simulink model "Six_DOF"  (R2018b)
settings: Solver=FixedStepAuto  StartTime=0.0  StopTime=1000  FixedStep=1/90  MaxStep=2.0  RelTol=1e-3
InitFcn:
  | initializeVariables
StopFcn:
  | postProcessResults
values from neighbouring files (symbols this model uses):
  airplane =     [Airplane.mat]    (also in POC_airplane.mat; POC_test.mat; calculateForces.m = A.airplane; cl_test2.m = A.airplane)
  m = 3000    [InerGeo.mat]    (also in calculateForces.m = [Cl;Cm;Cn]*(0.5*rho*Vinf^2*S*cbar); initializeVariables.m = airplane.weights.MTOW)
undefined symbols (not defined in the file or in its folder): ft, s
libraries: simulink_extras x14, aerolibconvert2 x5, simulink x5, aerolibasang x4, aerolibanimutils x2, shared6dof x1, aerolibfltsims x1, dspstat3 x1
settings Model: Creator=Devansh  LastModifiedBy=jmzg1
settings DebuggingCC: ReadBeforeWriteMsg=DisableAll  WriteAfterWriteMsg=DisableAll  WriteAfterReadMsg=DisableAll  MultiTaskDSMMsg=none
settings HardwareCC: ProdBitPerLong=64  ProdHWDeviceType=Intel->x86-64 (Mac OS X)
settings ModelReferenceCC: UpdateModelReferenceTargets=IfOutOfDate
settings SFSimCC: SFSimEcho=off  SimUseLocalCustomCode=off
settings RTWCC: RTWUseLocalCustomCode=off
settings CodeAppCC: StateflowObjectComments=on

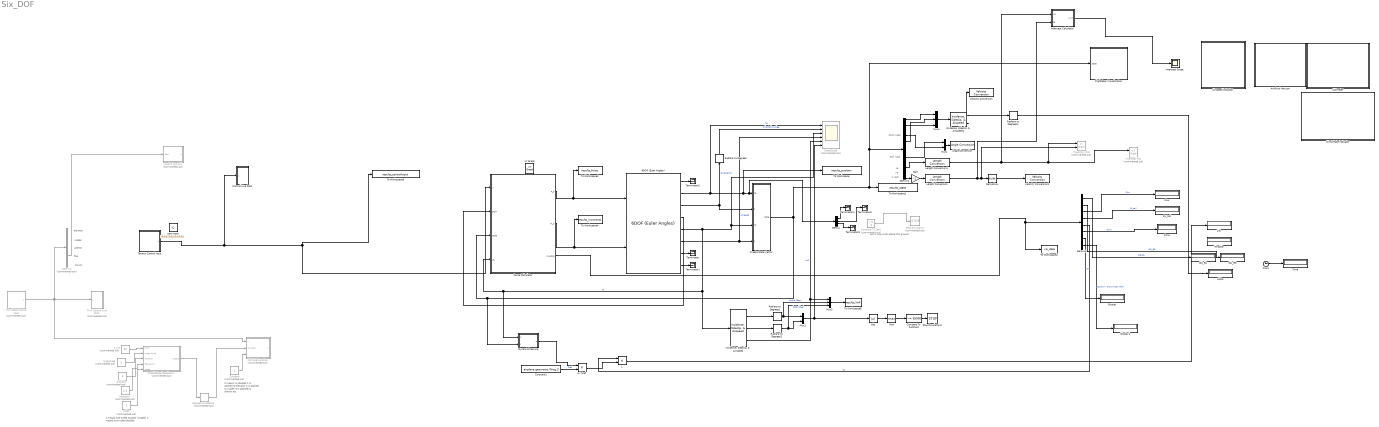
== system Six_DOF ==
  note: Don't stop when plane hits ground
  note: ye
  note: xe
  note: Pitch (rad)
  note: Roll (rad)
  note: -z (alt)
  note: 0 means no doublet
      | 1 is applied to elevator
      | 2 is applied to rudder
      | 3 is applied to aileron
      | etc
  note: 1 means one-sided doublet (singlet)
      | 2 means two-sided doublet
  note: elevator
  note: thrust
  note: aileron
  note: flap
  note: rudder
  6DOF (Euler Angles) : shared6dof/6DOF (Euler Angles)  units=Metric (MKS)  mtype=Fixed  rep=Euler Angles  xme_0=initial_position  Vm_0=initial_velocity  eul_0=initial_orientation  pm_0=initial_rotation_rate  mass_0=m  mass_e=0.5  mass_f=2.0  inertia=inertia_matrix  inertia_e=eye(3)  inertia_f=2*eye(3)  k_quat=1.0  vre_flag=on  abi_flag=off  aMode=aMode  xme_statename=''  Vm_statename=''  eul_statename=''  quat_statename=''  pm_statename=''  mass_statename=''
      settings: SourceProductBaseCode=AE
  Abs : Abs
  Airspeed Indicator : Subsystem  DialogController=aeroblksHMICreateDDGDialog  IsWebBlock=on  mask(MWDashboardBlock){webBlockId=8d9783d0-213f-431d-81d5-df6f8443250f, webBlockType=airspeedindicator, ShowInLibBrowser=on, ShowInitialText=on, HMISrcModelName=Six_DOF}
      mask prompts: webBlockId "WebBlock Id"; webBlockType "WebBlock Type"; HMISrcModelName "Source Model"
      mask help: aeroblksHMI:aeroblkhmi:AirspeedIndicatorDialogDesc
      mask Help: eval('asbhmihelp(''airspeedindicator'')');
      mask Display:
      | if strcmp(get_param(bdroot(gcb),'BlockDiagramType'), 'library')
      |  image([(matlabroot) '/toolbox/aeroblks/aeroblks/hmi/icons/AirspeedIndicatorIcon.svg'])
      | end
  Alpha : Display
  Altimeter : Subsystem  DialogController=aeroblksHMICreateDDGDialog  IsWebBlock=on  mask(MWDashboardBlock){webBlockId=6144597a-42d7-4879-8f21-486f6f9b2aa0, webBlockType=altimeter, ShowInLibBrowser=on, ShowInitialText=on, HMISrcModelName=Six_DOF}
      mask prompts: webBlockId "WebBlock Id"; webBlockType "WebBlock Type"; HMISrcModelName "Source Model"
      mask help: aeroblksHMI:aeroblkhmi:AltimeterDialogDesc
      mask Help: eval('asbhmihelp(''altimeter'')');
      mask Display:
      | if strcmp(get_param(bdroot(gcb),'BlockDiagramType'), 'library')
      |  image([(matlabroot) '/toolbox/aeroblks/aeroblks/hmi/icons/AltimeterIcon.svg'])
      | end
  Angle Conversion : aerolibconvert2/Angle Conversion  IU=rad  OU=deg
  Artificial Horizon : Subsystem  DialogController=aeroblksHMICreateDDGDialog  IsWebBlock=on  mask(MWDashboardBlock){webBlockId=38a41c5b-4fd5-43b0-81e3-0962c7372bed, webBlockType=artificialhorizon, ShowInLibBrowser=on, ShowInitialText=on, HMISrcModelName=Six_DOF}
      mask prompts: webBlockId "WebBlock Id"; webBlockType "WebBlock Type"; HMISrcModelName "Source Model"
      mask help: aeroblksHMI:aeroblkhmi:ArtificialHorizonDialogDesc
      mask Help: eval('asbhmihelp(''artificialhorizon'')');
      mask Display:
      | if strcmp(get_param(bdroot(gcb),'BlockDiagramType'), 'library')
      |  image([(matlabroot) '/toolbox/aeroblks/aeroblks/hmi/icons/ArtificialHorizonIcon.svg'])
      | end
  CL_tail : Display
  CLw : Display
  Climb Rate Indicator : Subsystem  DialogController=aeroblksHMICreateDDGDialog  IsWebBlock=on  mask(MWDashboardBlock){webBlockId=32d20416-f2f6-4150-907f-86e68601f2fe, webBlockType=climbindicator, ShowInLibBrowser=on, ShowInitialText=on, HMISrcModelName=Six_DOF}
      mask prompts: webBlockId "WebBlock Id"; webBlockType "WebBlock Type"; HMISrcModelName "Source Model"
      mask help: aeroblksHMI:aeroblkhmi:ClimbIndicatorDialogDesc
      mask Help: eval('asbhmihelp(''climbindicator'')');
      mask Display:
      | if strcmp(get_param(bdroot(gcb),'BlockDiagramType'), 'library')
      |  image([(matlabroot) '/toolbox/aeroblks/aeroblks/hmi/icons/ClimbIndicatorIcon.svg'])
      | end
  Clock : Clock
  Cmw : Display
  Compare To Constant : simulink/Logic and Bit Operations/Compare To Constant  relop=>=  const=95000  OutDataTypeStr=boolean
  Compare To Zero : simulink/Logic and Bit Operations/Compare To Zero  Commented=on  relop=>=  OutDataTypeStr=boolean
  Constant : Constant  Commented=on
  Constant1 : Constant  Value=airplane.geometry.Wing.S
  Control Live Dials : Subsystem
  Create State Vector : Subsystem
  Degrees to Radians : simulink_extras/Transformations/Degrees to Radians  Commented=on
  Demux : Demux  Outputs=3
  Demux1 : Demux  Outputs=12
  Demux2 : Demux  Commented=on  Outputs=[1 1 1 2 4]
  Demux3 : Demux  Outputs=8
  Derivative : Derivative
  Display : Display
  Display1 : Display
  DynamicPressure : MATLAB Function  TreatAsAtomicUnit=on
  FlightGear Visualization : Subsystem
  Force Calculator : Subsystem
  Gain : Gain  Gain=-1
  "Incidence, Sideslip, & Airspeed" : aerolibasang/Incidence, Sideslip, & Airspeed
      settings: SourceProductName=Aerospace Blockset
  "Incidence, Sideslip, & Airspeed1" : aerolibasang/Incidence, Sideslip, & Airspeed
      settings: SourceProductName=Aerospace Blockset
  Intercept Calculator : Subsystem
  Intercept Plot : simulink/Sinks/XY Graph  Commented=on  xmin=-1  xmax=1  ymin=-1  ymax=1  st=-1
  Intercept Scope : Scope
  L : Product
  Length Conversion : aerolibconvert2/Length Conversion  IU=m  OU=ft
  Length Conversion1 : aerolibconvert2/Length Conversion  IU=m  OU=ft
  Lift : Display
  MATLAB Function : MATLAB Function  Commented=on  TreatAsAtomicUnit=on
  Max : MinMax  Function=max
  Mux1 : Mux  Inputs=2
  Mux2 : Mux  Inputs=2
  Mux3 : Mux  Inputs=3
  Mux4 : Mux  Inputs=3
  Radians to Degrees{,1..2,4} (4 alike) : simulink_extras/Transformations/Radians to Degrees
  Scott's Joystick : Subsystem  Commented=on
  "StateScope " : Scope  Commented=on  NumInputPorts=6
  Stop Simulation : Stop  Commented=on
  Stop Simulation1 : Stop
  Taranis Control Input : Subsystem
  Terminator{,1..5} (6 alike) : Terminator
  Throttle : Display
  Time : Display
  To Workspace : ToWorkspace  VariableName=results_position  SaveFormat=Timeseries  SampleTime=-1
  To Workspace1 : ToWorkspace  VariableName=results_state  SaveFormat=Timeseries  SampleTime=-1
  To Workspace2 : ToWorkspace  VariableName=vis_data  SaveFormat=Timeseries  SampleTime=-1
  To Workspace3 : ToWorkspace  VariableName=results_force  SaveFormat=Timeseries  SampleTime=-1
  To Workspace4 : ToWorkspace  VariableName=results_moments  SaveFormat=Timeseries  SampleTime=-1
  To Workspace5 : ToWorkspace  VariableName=results_controlinput  SaveFormat=Timeseries  SampleTime=-1
  To Workspace6 : ToWorkspace  VariableName=results_Vinf  SaveFormat=Timeseries  SampleTime=-1
  Trajectory Plot : simulink/Sinks/XY Graph  Commented=on  xmin=0  xmax=10000  ymin=2950  ymax=3050  st=-1
  Trim Control Live Dials : Subsystem  Commented=on
  Trim State Control Input : Subsystem  Commented=on
  Velocity Conversion : aerolibconvert2/Velocity Conversion  IU=m/s  OU=kts
  Velocity Conversion1 : aerolibconvert2/Velocity Conversion  IU=ft/s  OU=ft/min
  dCJ_BL : Display
  dCJ_BR : Display
  duration : Constant  Commented=on  Value=4
  frequency : Constant  Commented=on  Value=1/4  OutDataTypeStr=Inherit: Inherit via back propagation
  magnitude : Constant  Commented=on  Value=3
  oneSideStepUpandDown : Subsystem  Commented=on
  q * Sref : Product
  sides : Constant  Commented=on  Value=2  OutDataTypeStr=Inherit: Inherit via back propagation
  t_crit : Constant  Commented=on  Value=32
  zero input : Constant  Value=[0;0;0;[0;0];[0;0;0;0]]
  XY Graph : simulink/Sinks/XY Graph  IOType=viewer  xmin=0  xmax=1000  ymin=900  ymax=1000  st=-1
  wires:
  6DOF (Euler Angles)/2 -> "StateScope "/1, To Workspace/1, Demux/1, Create State Vector/1(Xe)  "Xe"
  6DOF (Euler Angles)/3 -> Create State Vector/2(orientation), Radians to Degrees/1  "Orientation"
  6DOF (Euler Angles)/5 -> "StateScope "/3, Create State Vector/3(Vb), DynamicPressure/1(V), Force Calculator/4(Vb), "Incidence, Sideslip, & Airspeed"/1  "Vb"
  6DOF (Euler Angles)/6 -> "StateScope "/4, Create State Vector/4(omega b)  "omegab"
  "Incidence, Sideslip, & Airspeed"/3 -> Mux3/1, "StateScope "/5  "Vinf"
  "Incidence, Sideslip, & Airspeed"/1 -> Radians to Degrees1/1
  "Incidence, Sideslip, & Airspeed"/2 -> Radians to Degrees2/1
  Radians to Degrees/1 -> "StateScope "/2  "orientation_deg"
  Radians to Degrees1/1 -> Mux3/2, Mux2/1  "alpha (deg)"
  Radians to Degrees2/1 -> Mux3/3, Mux2/2  "beta (deg)"
  6DOF (Euler Angles)/7 -> Terminator/1
  6DOF (Euler Angles)/8 -> Terminator1/1
  6DOF (Euler Angles)/1 -> Terminator2/1
  t_crit/1 -> oneSideStepUpandDown/1(t_crit)
  magnitude/1 -> oneSideStepUpandDown/2(magnitude)
  duration/1 -> oneSideStepUpandDown/3(duration)
  oneSideStepUpandDown/1(output) -> Degrees to Radians/1
  Create State Vector/1(state) -> DynamicPressure/2(x), Force Calculator/3(state), FlightGear Visualization/1(state), Demux1/1, To Workspace1/1
  Mux3/1 -> To Workspace6/1
  Compare To Zero/1 -> Stop Simulation/1
  Degrees to Radians/1 -> MATLAB Function/2(doublet)
  Demux/1 -> Terminator4/1
  Demux/2 -> Terminator5/1
  Mux2/1 -> Abs/1, "StateScope "/6
  Abs/1 -> Max/1
  Max/1 -> Compare To Constant/1
  Compare To Constant/1 -> Stop Simulation1/1
  Constant/1 -> MATLAB Function/3(i)
  Force Calculator/1(F_b) -> 6DOF (Euler Angles)/1, To Workspace3/1
  Force Calculator/2(M_b) -> 6DOF (Euler Angles)/2, To Workspace4/1
  6DOF (Euler Angles)/4 -> Force Calculator/2(DCM)
  Demux1/12 -> Gain/1
  Gain/1 -> Length Conversion/1
  Demux1/4 -> Mux1/2
  Demux1/8 -> Mux1/1
  Mux1/1 -> Angle Conversion/1
  Demux1/1 -> Mux4/1
  Demux1/5 -> Mux4/2
  Demux1/2 -> Mux4/3
  Mux4/1 -> "Incidence, Sideslip, & Airspeed1"/1
  "Incidence, Sideslip, & Airspeed1"/3 -> Velocity Conversion/1
  Length Conversion/1 -> Intercept Calculator/2(ze), Trajectory Plot/2, Derivative/1
  Derivative/1 -> Velocity Conversion1/1
  DynamicPressure/1(q) -> q * Sref/1
  Constant1/1 -> q * Sref/2  "Sref"
  q * Sref/1 -> L/2
  L/1 -> Lift/1
  "Incidence, Sideslip, & Airspeed1"/1 -> Radians to Degrees4/1
  Radians to Degrees4/1 -> Alpha/1
  Force Calculator/3(vis_data) -> To Workspace2/1, Demux3/1
  Demux3/1 -> dCJ_BL/1  "dCJ_BL"
  Demux3/2 -> dCJ_BR/1  "dCJ_BR"
  Demux3/3 -> CLw/1  "CLw"
  Demux3/4 -> CL_tail/1  "CL_tail"
  Demux3/5 -> L/1  "CL"
  Demux3/6 -> Cmw/1  "Cmw"
  Demux1/10 -> Length Conversion1/1
  Length Conversion1/1 -> Intercept Calculator/1(xe), Intercept Plot/1, Trajectory Plot/1
  Taranis Control Input/1(u) -> Control Live Dials/1(u), Force Calculator/1(u), To Workspace5/1
  Intercept Calculator/1(x-int) -> Intercept Scope/1
  Clock/1 -> Time/1
  frequency/1 -> oneSideStepUpandDown/4(frequency)
  sides/1 -> oneSideStepUpandDown/5(sides)
  Trim State Control Input/1(u) -> Trim Control Live Dials/1(u), MATLAB Function/1(u), Demux2/1
  Demux2/4 -> Scott's Joystick/1(flap)
  Demux/3 -> Terminator3/1
  Demux3/7 -> Display/1  "CX"
  Demux3/8 -> Display1/1  "Epsilon / Downwash (rad)"

== system Six_DOF/Airspeed Indicator ==

== system Six_DOF/Altimeter ==

== system Six_DOF/Artificial Horizon ==

== system Six_DOF/Climb Rate Indicator ==

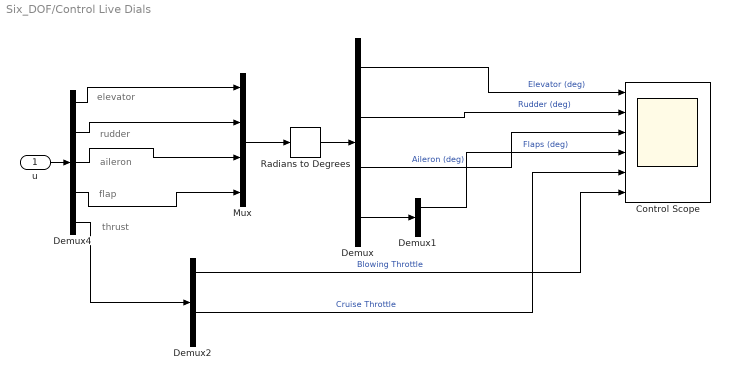
== system Six_DOF/Control Live Dials ==
  note: elevator
  note: thrust
  note: rudder
  note: aileron
  note: flap
  u : Inport
  Control Scope : Scope  NumInputPorts=6
  Demux : Demux  Outputs=[1,1,1,2]
  Demux1 : Demux  Outputs=2
  Demux2 : Demux
  Demux4 : Demux  Outputs=[1 1 1 2 4]
  Mux : Mux
  Radians to Degrees : simulink_extras/Transformations/Radians to Degrees
  wires:
  Demux4/3 -> Mux/3
  Demux4/2 -> Mux/2
  u/1 -> Demux4/1
  Demux4/1 -> Mux/1
  Demux4/4 -> Mux/4
  Demux4/5 -> Demux2/1
  Mux/1 -> Radians to Degrees/1
  Radians to Degrees/1 -> Demux/1
  Demux/1 -> Control Scope/1  "Elevator (deg)"
  Demux/2 -> Control Scope/2  "Rudder (deg)"
  Demux/3 -> Control Scope/3  "Aileron (deg)"
  Demux/4 -> Demux1/1
  Demux1/1 -> Control Scope/4  "Flaps (deg)"
  Demux2/1 -> Control Scope/6  "Blowing Throttle"
  Demux2/3 -> Control Scope/5  "Cruise Throttle"

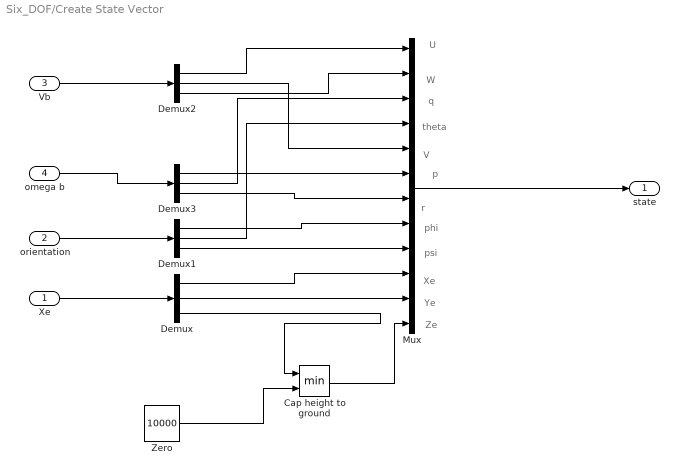
== system Six_DOF/Create State Vector ==
  note: Ze
  note: Ye
  note: Xe
  note: psi
  note: phi
  note: r
  note: p
  note: V
  note: theta
  note: q
  note: W
  note: U
  Xe : Inport
  orientation : Inport  Port=2
  Vb : Inport  Port=3
  omega b : Inport  Port=4
  Cap height to ground : MinMax  Inputs=2
  Demux{,1..3} (4 alike) : Demux  Outputs=3
  Mux : Mux  Inputs=12
  Zero : Constant  Value=10000  OutDataTypeStr=Inherit: Inherit via back propagation
  state : Outport
  wires:
  Demux2/1 -> Mux/1
  Demux2/2 -> Mux/5
  Vb/1 -> Demux2/1
  Demux1/1 -> Mux/8
  Demux/1 -> Mux/10
  Demux/3 -> Cap height to ground/1
  Xe/1 -> Demux/1
  orientation/1 -> Demux1/1
  Mux/1 -> state/1
  Demux3/1 -> Mux/6
  Demux1/3 -> Mux/9
  Demux/2 -> Mux/11
  Demux3/2 -> Mux/3
  Demux1/2 -> Mux/4
  Demux2/3 -> Mux/2
  Demux3/3 -> Mux/7
  omega b/1 -> Demux3/1
  Cap height to ground/1 -> Mux/12
  Zero/1 -> Cap height to ground/2

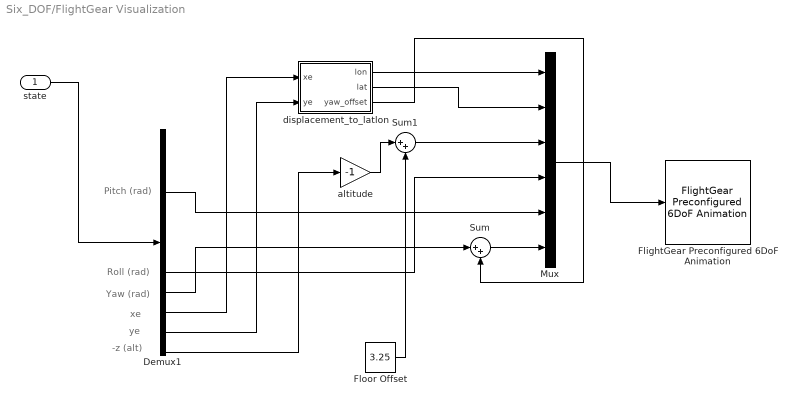
== system Six_DOF/FlightGear Visualization ==
  note: Yaw (rad)
  note: xe
  note: Pitch (rad)
  note: Roll (rad)
  note: ye
  note: -z (alt)
  state : Inport
  Demux1 : Demux  Outputs=12
  FlightGear Preconfigured 6DoF Animation : aerolibfltsims/FlightGear Preconfigured 6DoF Animation  xFlightGearVersion=v2018.1  DestinationIpAddress=127.0.0.1  DestinationPort=5502  SampleTime=-1  packetVersion=24
      settings: SourceProductName=Aerospace Blockset
  Floor Offset : Constant  Value=3.25  OutDataTypeStr=Inherit: Inherit via back propagation
  Mux : Mux  Inputs=6
  Sum : Sum  Inputs=|++
  Sum1 : Sum  Inputs=|++
  altitude : Gain  Gain=-1
  displacement_to_latlon : MATLAB Function  TreatAsAtomicUnit=on
  wires:
  Demux1/10 -> displacement_to_latlon/1(xe)
  Demux1/11 -> displacement_to_latlon/2(ye)
  displacement_to_latlon/1(lon) -> Mux/1
  displacement_to_latlon/2(lat) -> Mux/2
  state/1 -> Demux1/1
  Demux1/12 -> altitude/1
  Demux1/4 -> Mux/5
  Demux1/8 -> Mux/4
  Mux/1 -> FlightGear Preconfigured 6DoF Animation/1
  displacement_to_latlon/3(yaw_offset) -> Sum/2
  Sum/1 -> Mux/6
  Demux1/9 -> Sum/1
  altitude/1 -> Sum1/1
  Floor Offset/1 -> Sum1/2
  Sum1/1 -> Mux/3

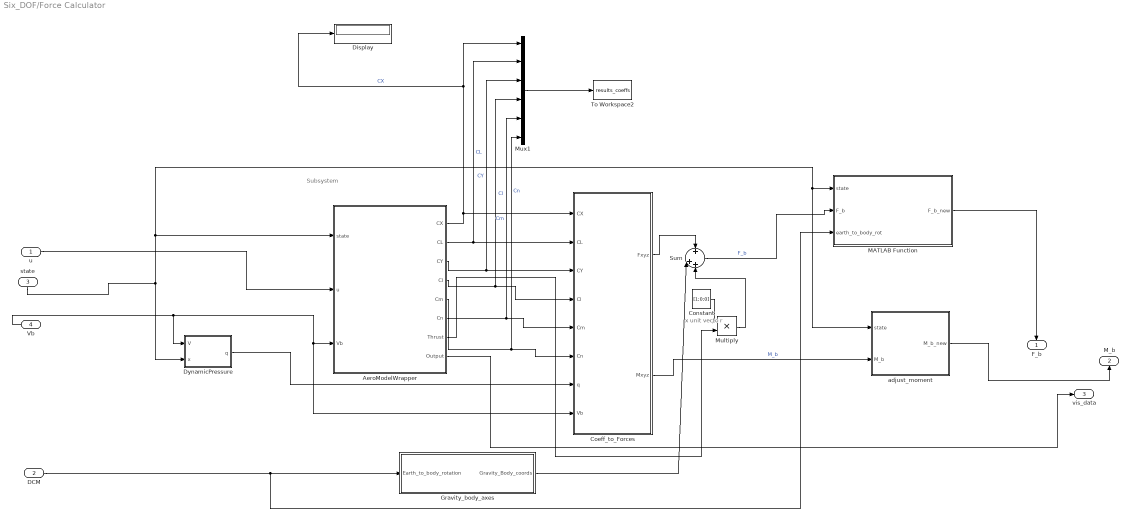
== system Six_DOF/Force Calculator ==
  note: x unit vecto
      | r
  note: Subsystem
  u : Inport
  DCM : Inport  Port=2
  state : Inport  Port=3
  Vb : Inport  Port=4
  AeroModelWrapper : Subsystem
  Coeff_to_Forces : Subsystem  TreatAsAtomicUnit=on
  Constant : Constant  Value=[1;0;0]
  Display : Display
  DynamicPressure : MATLAB Function  TreatAsAtomicUnit=on
  Gravity_body_axes : Subsystem
  MATLAB Function : MATLAB Function  TreatAsAtomicUnit=on
  Multiply : Product
  Mux1 : Mux  Inputs=6
  Sum : Sum  Inputs=+|++
  To Workspace2 : ToWorkspace  VariableName=results_coeffs  SaveFormat=Timeseries  SampleTime=-1
  adjust_moment : MATLAB Function  TreatAsAtomicUnit=on
  F_b : Outport
  M_b : Outport  Port=2
  vis_data : Outport  Port=3
  wires:
  Mux1/1 -> To Workspace2/1
  DCM/1 -> MATLAB Function/3(earth_to_body_rot), Gravity_body_axes/1(Earth_to_body_rotation)
  u/1 -> AeroModelWrapper/2(u)
  state/1 -> adjust_moment/1(state), MATLAB Function/1(state), AeroModelWrapper/1(state), DynamicPressure/2(x)
  Vb/1 -> Coeff_to_Forces/8(Vb), AeroModelWrapper/3(Vb), DynamicPressure/1(V)
  Gravity_body_axes/1(Gravity_Body_coords) -> Sum/2
  Sum/1 -> MATLAB Function/2(F_b)  "F_b"
  Coeff_to_Forces/1(Fxyz) -> Sum/1
  DynamicPressure/1(q) -> Coeff_to_Forces/7(q)
  Coeff_to_Forces/2(Mxyz) -> adjust_moment/2(M_b)  "M_b"
  AeroModelWrapper/6(Cn) -> Coeff_to_Forces/6(Cn), Mux1/6  "Cn"
  AeroModelWrapper/5(Cm) -> Coeff_to_Forces/5(Cm), Mux1/5  "Cm"
  AeroModelWrapper/4(Cl) -> Coeff_to_Forces/4(Cl), Mux1/4  "Cl"
  AeroModelWrapper/2(CL) -> Mux1/2, Coeff_to_Forces/2(CL)  "CL"
  AeroModelWrapper/3(CY) -> Mux1/3, Coeff_to_Forces/3(CY)  "CY"
  AeroModelWrapper/1(CX) -> Mux1/1, Display/1, Coeff_to_Forces/1(CX)  "CX"
  AeroModelWrapper/8(Output) -> vis_data/1
  MATLAB Function/1(F_b_new) -> F_b/1
  adjust_moment/1(M_b_new) -> M_b/1
  AeroModelWrapper/7(Thrust) -> Multiply/2
  Constant/1 -> Multiply/1
  Multiply/1 -> Sum/3

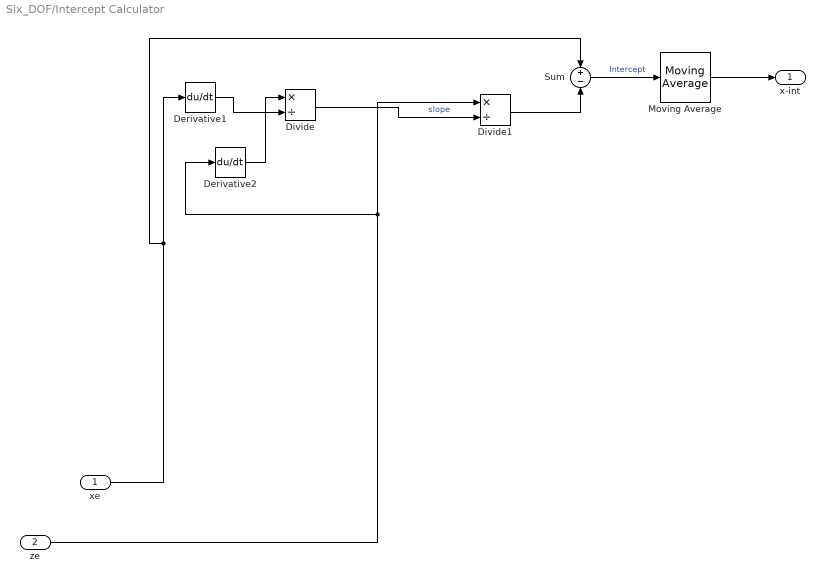
== system Six_DOF/Intercept Calculator ==
  xe : Inport
  ze : Inport  Port=2
  Derivative1 : Derivative
  Derivative2 : Derivative
  Divide : Product  Inputs=*/
  Divide1 : Product  Inputs=*/
  Moving Average : dspstat3/Moving Average  Method=Sliding window  ForgettingFactorPort=off  SpecifyWindowLength=on  WindowLength=10  ForgettingFactor=0.9  SimulateUsing=Code generation
  Sum : Sum  Inputs=+-
  x-int : Outport
  wires:
  Derivative1/1 -> Divide/2
  Derivative2/1 -> Divide/1
  xe/1 -> Sum/1, Derivative1/1
  Sum/1 -> Moving Average/1  "Intercept"
  ze/1 -> Derivative2/1, Divide1/1
  Divide/1 -> Divide1/2  "slope"
  Divide1/1 -> Sum/2
  Moving Average/1 -> x-int/1

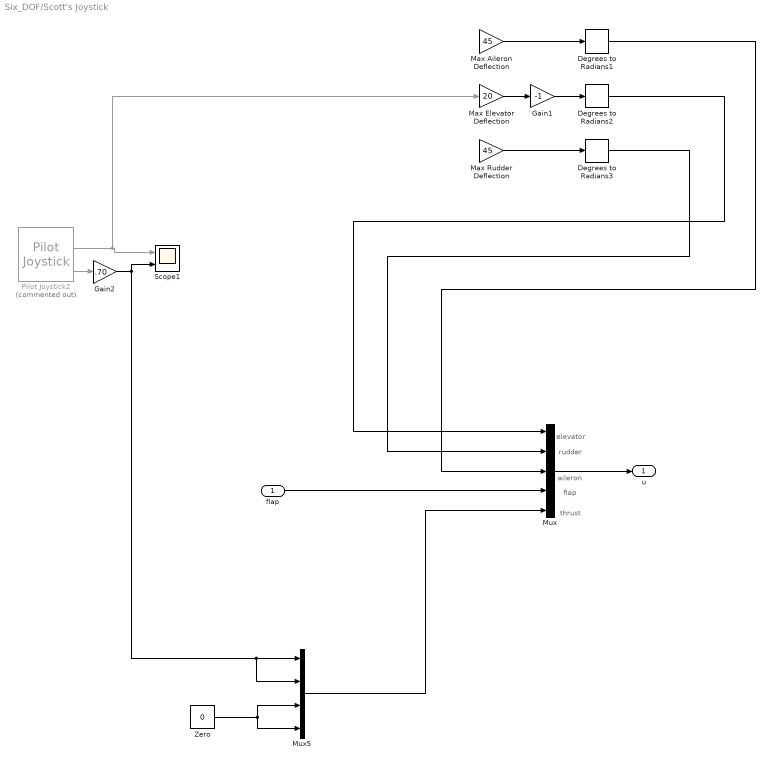
== system Six_DOF/Scott's Joystick ==
  note: thrust
  note: flap
  note: aileron
  note: rudder
  note: elevator
  flap : Inport
  Degrees to Radians1 : simulink_extras/Transformations/Degrees to Radians
  Degrees to Radians2 : simulink_extras/Transformations/Degrees to Radians
  Degrees to Radians3 : simulink_extras/Transformations/Degrees to Radians
  Gain1 : Gain  Gain=-1
  Gain2 : Gain  Gain=.70
  Max Aileron Deflection : Gain  Gain=45
  Max Elevator Deflection : Gain  Gain=20
  Max Rudder Deflection : Gain  Gain=45
  Mux : Mux  Inputs=5
  Mux5 : Mux
  Pilot Joystick2 : aerolibanimutils/Pilot Joystick  Commented=on  JoystickID=Joystick1  OutputConfiguration=FourAxis  SampleTime=1/30
  Scope1 : Scope  NumInputPorts=2
  Zero : Constant  Value=0  OutDataTypeStr=Inherit: Inherit via back propagation
  u : Outport
  wires:
  Max Elevator Deflection/1 -> Gain1/1
  ? -> Max Aileron Deflection/1
  Mux/1 -> u/1
  Pilot Joystick2/4 -> Gain2/1
  Gain2/1 -> Mux5/2, Mux5/1, Scope1/2
  Degrees to Radians1/1 -> Mux/3
  Zero/1 -> Mux5/4, Mux5/3
  flap/1 -> Mux/4
  Degrees to Radians3/1 -> Mux/2
  Degrees to Radians2/1 -> Mux/1
  Max Rudder Deflection/1 -> Degrees to Radians3/1
  Max Aileron Deflection/1 -> Degrees to Radians1/1
  Pilot Joystick2/2 -> Max Elevator Deflection/1, Scope1/1
  ? -> Max Rudder Deflection/1
  Gain1/1 -> Degrees to Radians2/1
  Mux5/1 -> Mux/5

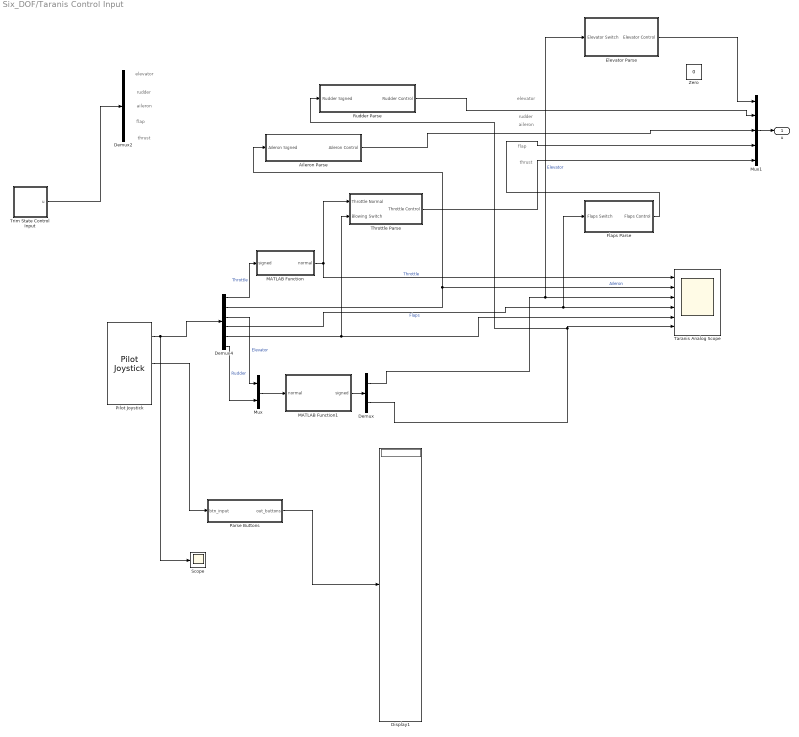
== system Six_DOF/Taranis Control Input ==
  note: rudder
  note: elevator
  note: thrust
  note: aileron
  note: flap
  note: flap
  note: thrust
  note: elevator
  note: rudder
  note: aileron
  Aileron Parse : Subsystem
  Demux : Demux  Outputs=2
  Demux2 : Demux  Outputs=[1 1 1 2 4]
  Demux4 : Demux  Outputs=6
  Display1 : Display
  Elevator Parse : Subsystem
  Flaps Parse : Subsystem
  MATLAB Function : MATLAB Function  TreatAsAtomicUnit=on
  MATLAB Function1 : MATLAB Function  TreatAsAtomicUnit=on
  Mux : Mux  Inputs=2
  Mux1 : Mux  Inputs=5
  Parse Buttons : MATLAB Function  TreatAsAtomicUnit=on
  Pilot Joystick : aerolibanimutils/Pilot Joystick  JoystickID=Joystick1  OutputConfiguration=AllOutputs  SampleTime=1/30
  Rudder Parse : Subsystem
  Scope : Scope
  Taranis Analog Scope : Scope  NumInputPorts=6
  Throttle Parse : Subsystem
  Trim State Control Input : Subsystem
  Zero : Constant  Value=0  OutDataTypeStr=Inherit: Inherit via back propagation
  u : Outport
  wires:
  Demux4/5 -> Throttle Parse/2(Blowing Switch), Taranis Analog Scope/5
  Demux4/1 -> MATLAB Function/1(signed)  "Throttle"
  Demux4/3 -> Mux/1  "Elevator"
  Demux4/6 -> Mux/2  "Rudder"
  Pilot Joystick/1 -> Scope/1, Demux4/1
  Demux4/4 -> Taranis Analog Scope/4, Flaps Parse/1(Flaps Switch)  "Flaps"
  Demux4/2 -> Taranis Analog Scope/2, Aileron Parse/1(Aileron Signed)  "Aileron"
  MATLAB Function/1(normal) -> Throttle Parse/1(Throttle Normal), Taranis Analog Scope/1  "Throttle"
  Mux/1 -> MATLAB Function1/1(normal)
  MATLAB Function1/1(signed) -> Demux/1
  Demux/1 -> Elevator Parse/1(Elevator Switch), Taranis Analog Scope/3  "Elevator"
  Trim State Control Input/1(u) -> Demux2/1
  Mux1/1 -> u/1
  Elevator Parse/1(Elevator Control) -> Mux1/1
  Pilot Joystick/2 -> Parse Buttons/1(btn_input)
  Parse Buttons/1(out_buttons) -> Display1/1
  Flaps Parse/1(Flaps Control) -> Mux1/4
  Demux/2 -> Rudder Parse/1(Rudder Signed), Taranis Analog Scope/6
  Rudder Parse/1(Rudder Control) -> Mux1/2
  Aileron Parse/1(Aileron Control) -> Mux1/3
  Throttle Parse/1(Throttle Control) -> Mux1/5

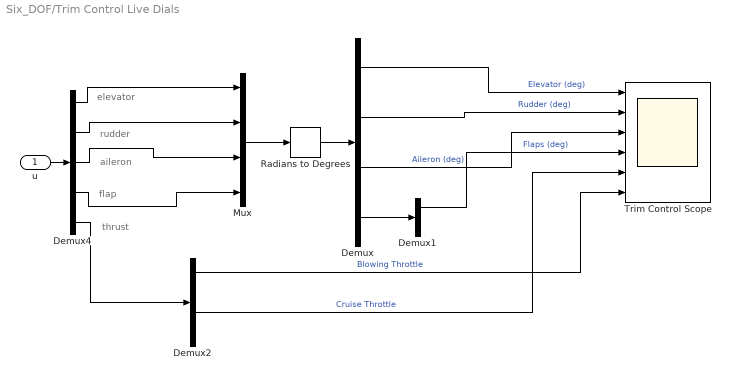
== system Six_DOF/Trim Control Live Dials ==
  note: elevator
  note: thrust
  note: rudder
  note: aileron
  note: flap
  u : Inport
  Demux : Demux  Outputs=[1,1,1,2]
  Demux1 : Demux  Outputs=2
  Demux2 : Demux
  Demux4 : Demux  Outputs=[1 1 1 2 4]
  Mux : Mux
  Radians to Degrees : simulink_extras/Transformations/Radians to Degrees
  Trim Control Scope : Scope  NumInputPorts=6
  wires:
  Demux4/3 -> Mux/3
  Demux4/2 -> Mux/2
  u/1 -> Demux4/1
  Demux4/1 -> Mux/1
  Demux4/4 -> Mux/4
  Demux4/5 -> Demux2/1
  Mux/1 -> Radians to Degrees/1
  Radians to Degrees/1 -> Demux/1
  Demux/1 -> Trim Control Scope/1  "Elevator (deg)"
  Demux/2 -> Trim Control Scope/2  "Rudder (deg)"
  Demux/3 -> Trim Control Scope/3  "Aileron (deg)"
  Demux/4 -> Demux1/1
  Demux1/1 -> Trim Control Scope/4  "Flaps (deg)"
  Demux2/1 -> Trim Control Scope/6  "Blowing Throttle"
  Demux2/3 -> Trim Control Scope/5  "Cruise Throttle"

== system Six_DOF/Trim State Control Input ==
  note: aileron
  note: flap
  note: thrust
  note: rudder
  note: elevator
  Aileron Angle : Constant  Value=u(3)
  Constant2 : Constant  Value=u(6:end)
  Elevator Angle : Constant  Value=u(1)
  Flap Angle : Constant  Value=u(4:5)
  Mux6 : Mux  Inputs=5
  Rudder Angle : Constant  Value=u(2)
  u : Outport
  wires:
  Mux6/1 -> u/1
  Rudder Angle/1 -> Mux6/2  "rudder"
  Flap Angle/1 -> Mux6/4  "flap"
  Aileron Angle/1 -> Mux6/3  "aileron"
  Elevator Angle/1 -> Mux6/1  "elevator"
  Constant2/1 -> Mux6/5  "thrust"

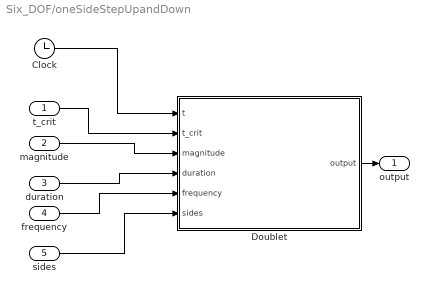
== system Six_DOF/oneSideStepUpandDown ==
  t_crit : Inport
  magnitude : Inport  Port=2
  duration : Inport  Port=3
  frequency : Inport  Port=4
  sides : Inport  Port=5
  Clock : Clock
      settings: Decimation=100
  Doublet : MATLAB Function  TreatAsAtomicUnit=on
  output : Outport
  wires:
  duration/1 -> Doublet/4(duration)
  t_crit/1 -> Doublet/2(t_crit)
  Doublet/1(output) -> output/1
  Clock/1 -> Doublet/1(t)
  magnitude/1 -> Doublet/3(magnitude)
  sides/1 -> Doublet/6(sides)
  frequency/1 -> Doublet/5(frequency)

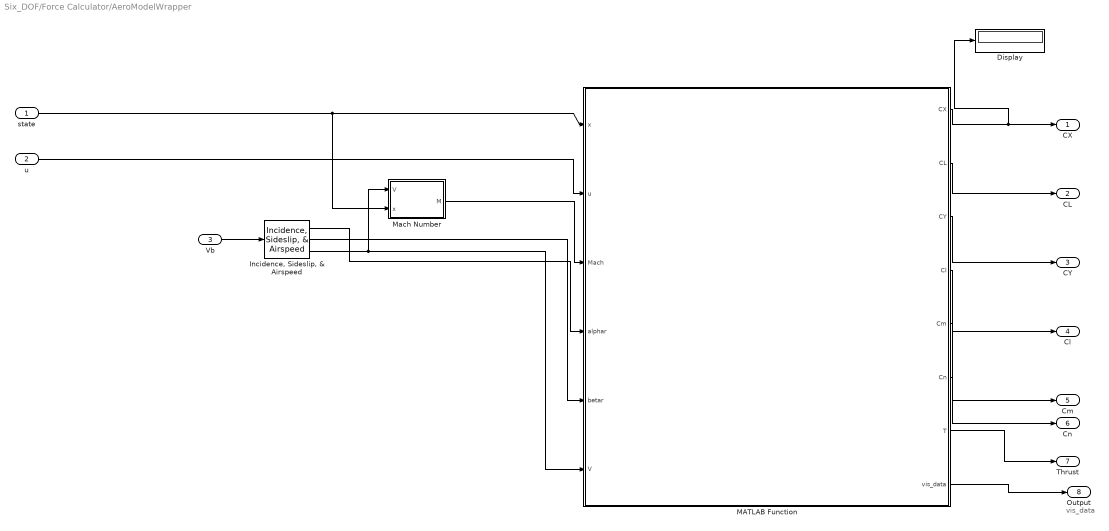
== system Six_DOF/Force Calculator/AeroModelWrapper ==
  note: vis_data
  state : Inport
  u : Inport  Port=2
  Vb : Inport  Port=3
  Display : Display
  "Incidence, Sideslip, & Airspeed" : aerolibasang/Incidence, Sideslip, & Airspeed
      settings: SourceProductName=Aerospace Blockset
  MATLAB Function : MATLAB Function  TreatAsAtomicUnit=on
  Mach Number : MATLAB Function  TreatAsAtomicUnit=on
  CX : Outport  OutDataTypeStr=double
  CL : Outport  Port=2  OutDataTypeStr=double
  CY : Outport  Port=3  OutDataTypeStr=double
  Cl : Outport  Port=4  OutDataTypeStr=double
  Cm : Outport  Port=5  OutDataTypeStr=double
  Cn : Outport  Port=6  OutDataTypeStr=double
  Thrust : Outport  Port=7
  Output : Outport  Port=8
  wires:
  MATLAB Function/1(CX) -> Display/1, CX/1
  MATLAB Function/2(CL) -> CL/1
  MATLAB Function/3(CY) -> CY/1
  MATLAB Function/4(Cl) -> Cl/1
  MATLAB Function/5(Cm) -> Cm/1
  MATLAB Function/6(Cn) -> Cn/1
  u/1 -> MATLAB Function/2(u)
  "Incidence, Sideslip, & Airspeed"/2 -> MATLAB Function/5(betar)
  "Incidence, Sideslip, & Airspeed"/1 -> MATLAB Function/4(alphar)
  "Incidence, Sideslip, & Airspeed"/3 -> Mach Number/1(V), MATLAB Function/6(V)
  Mach Number/1(M) -> MATLAB Function/3(Mach)
  Vb/1 -> "Incidence, Sideslip, & Airspeed"/1
  state/1 -> Mach Number/2(x), MATLAB Function/1(x)
  MATLAB Function/8(vis_data) -> Output/1
  MATLAB Function/7(T) -> Thrust/1

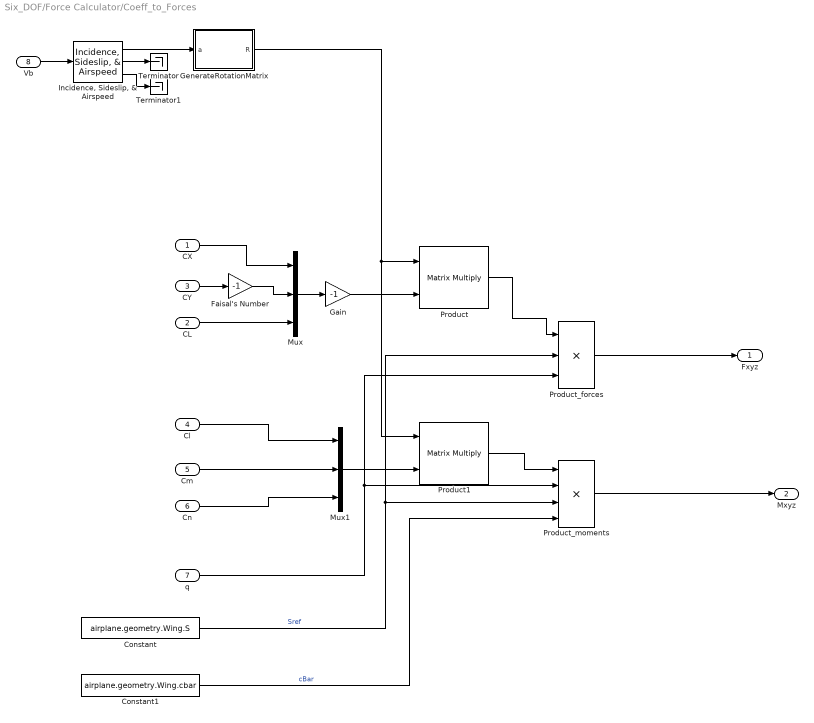
== system Six_DOF/Force Calculator/Coeff_to_Forces ==
  CX : Inport  OutDataTypeStr=double  PortDimensions=1
  CL : Inport  Port=2  OutDataTypeStr=double  PortDimensions=1
  CY : Inport  Port=3  OutDataTypeStr=double  PortDimensions=1
  Cl : Inport  Port=4  OutDataTypeStr=double  PortDimensions=1
  Cm : Inport  Port=5  OutDataTypeStr=double  PortDimensions=1
  Cn : Inport  Port=6  OutDataTypeStr=double  PortDimensions=1
  q : Inport  Port=7  OutDataTypeStr=double  PortDimensions=1
  Vb : Inport  Port=8  OutDataTypeStr=double  PortDimensions=3
  Constant : Constant  Value=airplane.geometry.Wing.S
  Constant1 : Constant  Value=airplane.geometry.Wing.cbar
  Faisal's Number : Gain  Gain=-1
  Gain : Gain  Gain=-1
  GenerateRotationMatrix : MATLAB Function  TreatAsAtomicUnit=on
  "Incidence, Sideslip, & Airspeed" : aerolibasang/Incidence, Sideslip, & Airspeed
      settings: SourceProductName=Aerospace Blockset
  Mux : Mux  Inputs=3
  Mux1 : Mux  Inputs=3
  Product : Product  Multiplication=Matrix(*)
  Product1 : Product  Multiplication=Matrix(*)
  Product_forces : Product  Inputs=3
  Product_moments : Product  Inputs=4
  Terminator : Terminator
  Terminator1 : Terminator
  Fxyz : Outport
  Mxyz : Outport  Port=2
  wires:
  CX/1 -> Mux/1
  CL/1 -> Mux/3
  Constant/1 -> Product_moments/3, Product_forces/2  "Sref"
  q/1 -> Product_forces/3, Product_moments/2
  Product_forces/1 -> Fxyz/1
  Cl/1 -> Mux1/1
  Cm/1 -> Mux1/2
  Cn/1 -> Mux1/3
  Constant1/1 -> Product_moments/4  "cBar"
  Product_moments/1 -> Mxyz/1
  Mux/1 -> Gain/1
  GenerateRotationMatrix/1(R) -> Product1/1, Product/1
  Product/1 -> Product_forces/1
  Vb/1 -> "Incidence, Sideslip, & Airspeed"/1
  "Incidence, Sideslip, & Airspeed"/1 -> GenerateRotationMatrix/1(a)
  "Incidence, Sideslip, & Airspeed"/2 -> Terminator/1
  "Incidence, Sideslip, & Airspeed"/3 -> Terminator1/1
  Mux1/1 -> Product1/2
  Product1/1 -> Product_moments/1
  Gain/1 -> Product/2
  CY/1 -> Faisal's Number/1
  Faisal's Number/1 -> Mux/2

== system Six_DOF/Force Calculator/Gravity_body_axes ==
  Earth_to_body_rotation : Inport
  Gravity Vector Earth Coords : Subsystem
  Product : Product  Multiplication=Matrix(*)
  Gravity_Body_coords : Outport
  wires:
  Earth_to_body_rotation/1 -> Product/1
  Gravity Vector Earth Coords/1("Gravity_vector_earth ") -> Product/2
  Product/1 -> Gravity_Body_coords/1

== system Six_DOF/Taranis Control Input/Aileron Parse ==
  Aileron Signed : Inport
  Cap Deflection : Subsystem
  Degrees to Radians : simulink_extras/Transformations/Degrees to Radians
  Gain1 : Gain  Gain=-1
  Max Aileron Deflection : Constant  Value=45  OutDataTypeStr=Inherit: Inherit via back propagation
  Multiply : Product
  Aileron Control : Outport
  wires:
  Aileron Signed/1 -> Gain1/1
  Gain1/1 -> Multiply/2  "Aileron"
  Multiply/1 -> Cap Deflection/1(Deflection)
  Max Aileron Deflection/1 -> Cap Deflection/2(Max Deflection), Multiply/1
  Cap Deflection/1(Capped) -> Degrees to Radians/1
  Degrees to Radians/1 -> Aileron Control/1

== system Six_DOF/Taranis Control Input/Elevator Parse ==
  Elevator Switch : Inport
  Cap Deflection : Subsystem
  Degrees to Radians : simulink_extras/Transformations/Degrees to Radians
  Display : Display
  Gain1 : Gain  Gain=-1
  Max Elevator Deflection (deg) : Constant  Value=20  OutDataTypeStr=Inherit: Inherit via back propagation
  Multiply1 : Product
  Elevator Control : Outport
  wires:
  Cap Deflection/1(Capped) -> Degrees to Radians/1, Display/1
  Max Elevator Deflection (deg)/1 -> Multiply1/1, Cap Deflection/2(Max Deflection)
  Gain1/1 -> Cap Deflection/1(Deflection)
  Elevator Switch/1 -> Multiply1/2
  Multiply1/1 -> Gain1/1
  Degrees to Radians/1 -> Elevator Control/1

== system Six_DOF/Taranis Control Input/Flaps Parse ==
  Flaps Switch : Inport
  Degrees to Radians : simulink_extras/Transformations/Degrees to Radians
  Display2 : Display
  Flap Angle (deg) : Display
  Max Flap Deflection (deg) : Constant  Value=70  OutDataTypeStr=Inherit: Inherit via back propagation
  Mux2 : Mux  Inputs=2
  flap_degrees : MATLAB Function  TreatAsAtomicUnit=on
  Flaps Control : Outport
  wires:
  Flaps Switch/1 -> flap_degrees/1(flap_switch), Display2/1
  flap_degrees/1(flap_angle) -> Degrees to Radians/1, Flap Angle (deg)/1
  Mux2/1 -> Flaps Control/1
  Degrees to Radians/1 -> Mux2/2, Mux2/1
  Max Flap Deflection (deg)/1 -> flap_degrees/2(max_def)

== system Six_DOF/Taranis Control Input/Rudder Parse ==
  Rudder Signed : Inport
  Cap Deflection : Subsystem
  Degrees to Radians : simulink_extras/Transformations/Degrees to Radians
  Gain1 : Gain  Gain=-1
  Max Rudder Deflection : Constant  Value=45  OutDataTypeStr=Inherit: Inherit via back propagation
  Multiply : Product
  Rudder Control : Outport
  wires:
  Rudder Signed/1 -> Gain1/1
  Gain1/1 -> Multiply/2  "Rudder"
  Multiply/1 -> Cap Deflection/1(Deflection)
  Max Rudder Deflection/1 -> Cap Deflection/2(Max Deflection), Multiply/1
  Cap Deflection/1(Capped) -> Degrees to Radians/1
  Degrees to Radians/1 -> Rudder Control/1

== system Six_DOF/Taranis Control Input/Throttle Parse ==
  Throttle Normal : Inport
  Blowing Switch : Inport  Port=2
  Blowing Parse : MATLAB Function  TreatAsAtomicUnit=on
  Display : Display
  Display1 : Display
  Mux5 : Mux
  Throttle Control : Outport
  wires:
  Mux5/1 -> Throttle Control/1  "Thrust"
  Blowing Switch/1 -> Blowing Parse/1(blow_switch)
  Throttle Normal/1 -> Mux5/3, Mux5/4, Display1/1
  Blowing Parse/1(blow_setting) -> Display/1, Mux5/2, Mux5/1

== system Six_DOF/Taranis Control Input/Trim State Control Input ==
  note: aileron
  note: flap
  note: thrust
  note: rudder
  note: elevator
  Aileron Angle : Constant  Value=u(3)
  Constant2 : Constant  Value=u(6:end)
  Elevator Angle : Constant  Value=u(1)
  Flap Angle : Constant  Value=u(4:5)
  Mux6 : Mux  Inputs=5
  Rudder Angle : Constant  Value=u(2)
  u : Outport
  wires:
  Mux6/1 -> u/1
  Rudder Angle/1 -> Mux6/2  "rudder"
  Flap Angle/1 -> Mux6/4  "flap"
  Aileron Angle/1 -> Mux6/3  "aileron"
  Elevator Angle/1 -> Mux6/1  "elevator"
  Constant2/1 -> Mux6/5  "thrust"

== system Six_DOF/Force Calculator/Gravity_body_axes/Gravity Vector Earth Coords ==
  Constant3 : Constant  Value=m
  Constant4 : Constant  Value=9.81
  Constant5 : Constant  Value=0
  Mux1 : Mux  Inputs=3
  gravitational force : Product
  "Gravity_vector_earth " : Outport
  wires:
  Constant4/1 -> gravitational force/2
  Constant3/1 -> gravitational force/1
  Constant5/1 -> Mux1/2, Mux1/1
  gravitational force/1 -> Mux1/3
  Mux1/1 -> "Gravity_vector_earth "/1

== system Six_DOF/Taranis Control Input/Aileron Parse/Cap Deflection ==
  Deflection : Inport
  Max Deflection : Inport  Port=2
  Min : MinMax  Inputs=2
  Multiply : Product
  Multiply2 : Product
  Sign : Signum
  Capped : Outport
  wires:
  Max Deflection/1 -> Min/2
  Deflection/1 -> Multiply/2, Sign/1
  Sign/1 -> Multiply2/1, Multiply/1
  Multiply/1 -> Min/1
  Multiply2/1 -> Capped/1
  Min/1 -> Multiply2/2

== system Six_DOF/Taranis Control Input/Elevator Parse/Cap Deflection ==
  Deflection : Inport
  Max Deflection : Inport  Port=2
  Min : MinMax  Inputs=2
  Multiply : Product
  Multiply2 : Product
  Sign : Signum
  Capped : Outport
  wires:
  Max Deflection/1 -> Min/2
  Deflection/1 -> Multiply/2, Sign/1
  Sign/1 -> Multiply2/1, Multiply/1
  Multiply/1 -> Min/1
  Multiply2/1 -> Capped/1
  Min/1 -> Multiply2/2

== system Six_DOF/Taranis Control Input/Rudder Parse/Cap Deflection ==
  Deflection : Inport
  Max Deflection : Inport  Port=2
  Min : MinMax  Inputs=2
  Multiply : Product
  Multiply2 : Product
  Sign : Signum
  Capped : Outport
  wires:
  Max Deflection/1 -> Min/2
  Deflection/1 -> Multiply/2, Sign/1
  Sign/1 -> Multiply2/1, Multiply/1
  Multiply/1 -> Min/1
  Multiply2/1 -> Capped/1
  Min/1 -> Multiply2/2

== matlab function Six_DOF/Force Calculator/DynamicPressure ==
  data: V input; q output; x input
function q = fcn(V,x)
%calculates the dynamic pressure using the flight speed and airspeed

h=-x(12); %extract the height

[~, ~, rho, ~, ~, ~, ~, ~] = int_std_atm(h);


q = 0.5*rho*norm(V)^2;


end

== matlab function Six_DOF/Force Calculator/AeroModelWrapper/MATLAB Function ==
  data: x input; u input; CX output; Mach input; alphar input; betar input; V input; CL output; CY output; Cl output; Cm output; Cn output; T output; vis_data output
	function [CX,CL,CY,Cl,Cm,Cn,T,vis_data] = AeroModelSSTOLSimulink(x,u,Mach,alphar,betar,V)
%	SSTOL Aero Model
%   x(1) = u_b          Body axis u velocity, m/s
%   x(2) = w_b          Body axis w velocity, m/s
%   x(3) = q            Pitch rate, rad/s
%   x(4) = theta        Pitch euler angle, rad
%   x(5) = v_b          Body axis v velocity, m/s
%   x(6) = p            Roll rate, rad/s
%   x(7) = r            Yaw rate, rad/s
%   x(8) = phi          Roll euler angle, rad
%   x(9) = psi          Yaw euler angle, rad
%   x(10) = xe          North position, Earth frame, m
%   x(11) = ye          East position, Earth frame, m
%   x(12) = ze =-h      Negative of altitude, Earth frame, m

%   u(1) = elevator deflection, rad, positive trailing edge down
%   u(2) = rudder deflection, rad, positive trailing edge down
%   u(3) = aileron deflection, rad, positive left trailing edge down
%   u(4) = left flap deflection, rad, positive trailing edge down
%   u(5) = right flap deflection, rad, positive trailing edge down
%   u(6:end) = u_t, thrust control vector, 0-1

%   u_thrust(1) = left blowing throttle, 0-1
%   u_thrust(2) = right blowing throttle, 0-1
%   u_thrust(3) = left thruster throttle, 0-1git
%   u_thrust(4) = right thruster throttle, 0-1

%	Inertial, Geometric, and Aerodynamic Properties
%   *** STOL_Input.m must first be run to save Airplane.mat***
	

    A=load('Airplane.mat');
    airplane=A.airplane;
    
    CX = 0;
    CL = 0;
    CY = 0;
    Cl = 0;
    Cm = 0;
    Cn = 0;
    T=0;
    [CX,CL,CY,Cl,Cm,Cn,T,vis_data] = AeroModelSSTOL(x,u,Mach,alphar,betar,V,airplane);

== matlab function Six_DOF/Force Calculator/AeroModelWrapper/Mach Number ==
  data: V input; M output; x input
function M = fcn(V,x)
%calculates the mach number

[~, ~, ~, a, ~, ~, ~, ~] = int_std_atm(-x(12));

M = norm(V)/a;

== matlab function Six_DOF/Force Calculator/Coeff_to_Forces/GenerateRotationMatrix ==
  data: a input; R output
function R = rotationMatrix(a)

R = [cos(a), 0, -sin(a); 0, 1, 0; sin(a), 0, cos(a)];

== matlab function Six_DOF/oneSideStepUpandDown/Doublet ==
  data: t input; output output; t_crit input; magnitude input; duration input; frequency input; sides input
function output = doublet(t,t_crit,magnitude,duration, frequency, sides)

% Outputs either a single or double sided doublet.
% The frequency argumnet applies only to the number of full double-sided
% doublets per second.

if (sides == 1) && (t > t_crit) && (t<(t_crit + duration))
    output = magnitude;
elseif (sides == 2) && (t > t_crit) && (t<(t_crit + duration))
    w = 2*pi*frequency;
    output = magnitude * sign(sin(w*(t-t_crit)));
elseif ~any(sides == [1 2])
    error("Number of doublet sides must be either 1 or 2");
else
    output = 0;
end

== matlab function Six_DOF/MATLAB Function ==
  data: u input; y output; doublet input; i input
function y = add_doublet(u, doublet, i)

y = u;

if i~=0
    y(i) = u(i)+doublet;
end

== matlab function Six_DOF/FlightGear Visualization/displacement_to_latlon ==
  data: lon output; xe input; lat output; ye input; yaw_offset output
function [lon,lat, yaw_offset] = fcn(xe, ye)

% Calculates latitude and longitude from linear displacement
% Input: displacement North (xe) and East (ye) in meters

% Initial latitude and longitude in radians

% PR
% lat0 = deg2rad(18.46327778);%deg2rad(42.37425);
% lon0 = deg2rad(-66.11083333);%deg2rad(-71.01789);

% Boston Logan
% lat0 = deg2rad(42.37425);
% lon0 = deg2rad(-71.01789);

% Plum Island
lat0 = deg2rad(42.79555556);
lon0 = deg2rad(-70.84583333);
runway_number = 8.5;

% Earth Radius (m)
R = 6378137;

% Calculate change from initial
dlat = xe / R;
dlon = ye / (R*cos(lat0));

% Offset for visual purposes / runway alignment
dlat_new = dlat*cosd(runway_number*10) - dlon*sind(runway_number*10);
dlon_new = dlat*sind(runway_number*10) + dlon*cosd(runway_number*10);

lat = rad2deg(lat0 + dlat_new);
lon = rad2deg(lon0 + dlon_new);
yaw_offset = deg2rad(runway_number*10);

== matlab function Six_DOF/DynamicPressure ==
  data: V input; q output; x input
function q = fcn(V,x)
%calculates the dynamic pressure using the flight speed and airspeed

h=-x(12); %extract the height

[~, ~, rho, ~, ~, ~, ~, ~] = int_std_atm(h);


q = 0.5*rho*norm(V)^2;


end

== matlab function Six_DOF/Taranis Control Input/MATLAB Function ==
  data: signed input; normal output
function normal = signed_to_normal(signed)

normal = (signed + 1) / 2;

== matlab function Six_DOF/Taranis Control Input/MATLAB Function1 ==
  data: normal input; signed output
function signed = normal_to_signed(normal)
% Converts 0 to 1 scale to -1 to +1
signed = 2*normal - 1;

== matlab function Six_DOF/Force Calculator/MATLAB Function ==
  data: state input; F_b input; F_b_new output; earth_to_body_rot input
function F_b_new = adjust_force(state, F_b, earth_to_body_rot)

h = state(12);
V_b=[state(1);state(5);state(2)];

if h < 0 % 6 in.
    F_b_new = F_b;
else
    body_to_earth_rot = earth_to_body_rot';
    F_e = body_to_earth_rot * F_b;
    V_e = body_to_earth_rot * V_b;
    %F_e(3) = min(0, F_e(3));
    k = 1000;
    d=50;
    d_x=1;
    %F_e(3) = F_e(3) + min(0, -k*h);
    F_e(3) = F_e(3) -k*h-d*V_e(3);
    F_e(2) = F_e(2)-d_x*V_e(2);
    F_e(1) = F_e(1)-d_x*V_e(1);
    F_b_new = earth_to_body_rot' * F_e;
    %F_b_new (1) = F_b_new(1) - d_x*V_b(1);
%end
end

== matlab function Six_DOF/Taranis Control Input/Parse Buttons ==
  data: btn_input input; out_buttons output
function out_buttons  = button_parse(btn_input)

in_bin = dec2bin(btn_input);

% Pad sizes
while length(in_bin) < 32
    in_bin = ['0', in_bin];
end

out_buttons = zeros(1,32) - 1;
for i=1:32
    if in_bin(i) == '0'
        out_buttons(i) == 0;
    elseif in_bin(i) == '1'
        out_buttons(i) == 1;
    end
end

== matlab function Six_DOF/Taranis Control Input/Flaps Parse/flap_degrees ==
  data: flap_switch input; flap_angle output; max_def input
function flap_angle = switch_flaps(flap_switch, max_def)
% Converts a switch input into a flap setting in degrees
% 
% flap_configs = [0, 20, 40]; % in degrees
% switch_configs = [1, 0, -1];
% 
% [~,switch_index] = min(abs(flap_switch - switch_configs));
% 
% flap_angle = flap_configs(switch_index);

% if flap_switch == -1
%     flap_angle = flap_configs(1);
% elseif flap_switch == 0
%     flap_angle = flap_configs(2);
% elseif flap_switch == 1
%     flap_angle = flap_configs(3);
% else
%     flap_angle = flap_switch;
% end

% Continuous flaps

flap_angle = max_def*(0.5*(flap_switch+1));

== matlab function Six_DOF/Taranis Control Input/Throttle Parse/Blowing Parse ==
  data: blow_switch input; blow_setting output
function blow_setting = blowing_parse(blow_switch)

blow_configs = [0, .30, .60];
switch_configs = [0, 0.5, 1];

[~,switch_index] = min(abs(blow_switch - switch_configs));

blow_setting = blow_configs(switch_index);

== matlab function Six_DOF/Force Calculator/adjust_moment ==
  data: state input; M_b_new output; M_b input
function M_b_new = adjust_moment(state, M_b)

h = state(12);

phi = state(8); % roll
theta = state(4); % pitch

p = state(6); % roll rate
q = state(3); % pitch rate
r = state(7); % yaw rate

if h < -0.2
    M_b_new = M_b;
else
    % k = torsional spring constants
    kphi = 160;
    ktheta = 200;
    
    % d = damping constants
    dphi = 20;
    dtheta = 20;
    dpsi= 20;
    
    dM_b_k = -[kphi*phi, ktheta*theta, 0]';
    dM_b_d = -[dphi*p, dtheta*q, dpsi*r]';
    M_b_new = M_b + dM_b_k + dM_b_d;
end
